simulink subsystem "PWM"  (R2024a)
settings: Solver=VariableStepAuto  StartTime=0.0  StopTime=10.0  RelTol=1e-3
libraries: simulink x1
settings Model: Creator=Peter  LastModifiedBy=Peter

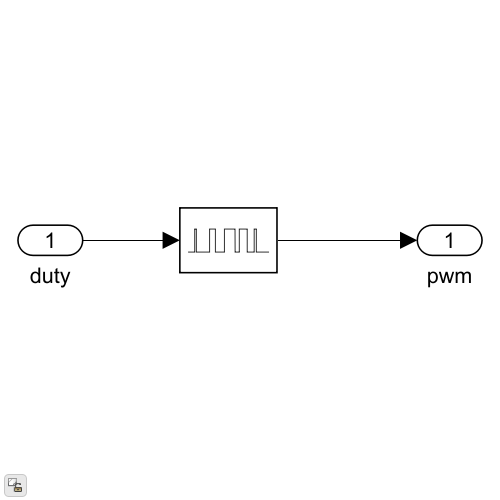
[thumbnail: Simulink's stored preview of the top-level diagram]
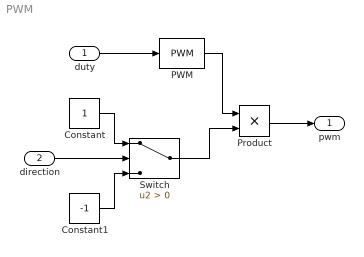
== system PWM ==
  duty : Inport
  direction : Inport  Port=2
  Constant : Constant
  Constant1 : Constant  Value=-1
  PWM : simulink/Discontinuities/PWM  DisableCoverage=on  Period=1e-5  InitialDelay=0  DisallowZeroDutyCycle=off  RunAtFixedTimeIntervals=off  SampleTime=0.1
  Product : Product
  Switch : Switch  Criteria=u2 > Threshold  SaturateOnIntegerOverflow=off  InputSameDT=off
  pwm : Outport
  wires:
  duty/1 -> PWM/1
  PWM/1 -> Product/1
  Switch/1 -> Product/2
  Product/1 -> pwm/1
  Constant1/1 -> Switch/3
  Constant/1 -> Switch/1
  direction/1 -> Switch/2
